simulink model "nonlinearSimulation"  (R2014a)
settings: Solver=ode4  StartTime=0.0  StopTime=50  FixedStep=.01  RelTol=1e-3
values from neighbouring files (symbols this model uses):
  C = [1 0 1 0]    [lQRdesign.m]    (also in state_space_design.m)
  g = 9.81    [energy_calc.m]    (also in lQRdesign.m; pendulum_eom.m; state_space_design.m)
  k1 = 1    [energy_calc.m]    (also in lQRdesign.m; pendulum_eom.m; state_space_design.m)
  k2 = 0.05    [energy_calc.m]    (also in lQRdesign.m; pendulum_eom.m; state_space_design.m)
  l = 1.2    [energy_calc.m]    (also in lQRdesign.m; pendulum_eom.m; state_space_design.m)
  M = 1.5    [energy_calc.m]    (also in lQRdesign.m; pendulum_eom.m; state_space_design.m)
  m = 0.5    [energy_calc.m]    (also in lQRdesign.m; pendulum_eom.m; state_space_design.m)
  sysKF = ss(A-Kf*C,[B Kf],eye(4),0*[B Kf])    [lQRdesign.m]
undefined symbols (not defined in the file or in its folder): Kr
settings Model: Creator=Mohamed Donia  LastModifiedBy=Mohamed Donia
settings DebuggingCC: AlgebraicLoopMsg=none

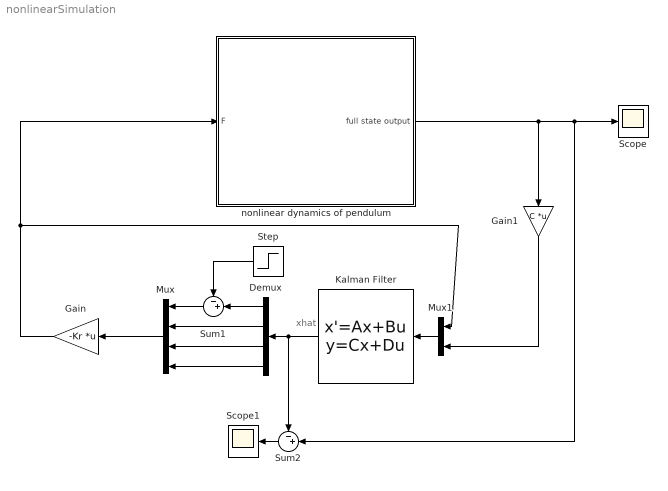
== system nonlinearSimulation ==
  note: xhat
  Demux : Demux
  Gain : Gain  Gain=-Kr  Multiplication=Matrix(K*u) (u vector)
  Gain1 : Gain  Gain=C  Multiplication=Matrix(K*u) (u vector)
  Kalman Filter : StateSpace  A=sysKF.A  B=sysKF.B  C=sysKF.C  D=sysKF.D  X0=[0 0 0 0]
  Mux : Mux
  Mux1 : Mux  Inputs=2
  Scope : Scope
  Scope1 : Scope
  Step : Step  Time=10  SampleTime=0
  Sum1 : Sum  Inputs=-+|
  Sum2 : Sum  Inputs=-+|
  nonlinear dynamics of pendulum : Subsystem
  wires:
  Kalman Filter/1 -> Sum2/1, Demux/1
  Demux/4 -> Mux/4
  Demux/3 -> Mux/3
  Demux/2 -> Mux/2
  Sum1/1 -> Mux/1
  Demux/1 -> Sum1/2
  Step/1 -> Sum1/1
  Mux/1 -> Gain/1
  Gain/1 -> nonlinear dynamics of pendulum/1(F), Mux1/1
  nonlinear dynamics of pendulum/1("full state output ") -> Sum2/2, Scope/1, Gain1/1
  Mux1/1 -> Kalman Filter/1
  Gain1/1 -> Mux1/2
  Sum2/1 -> Scope1/1

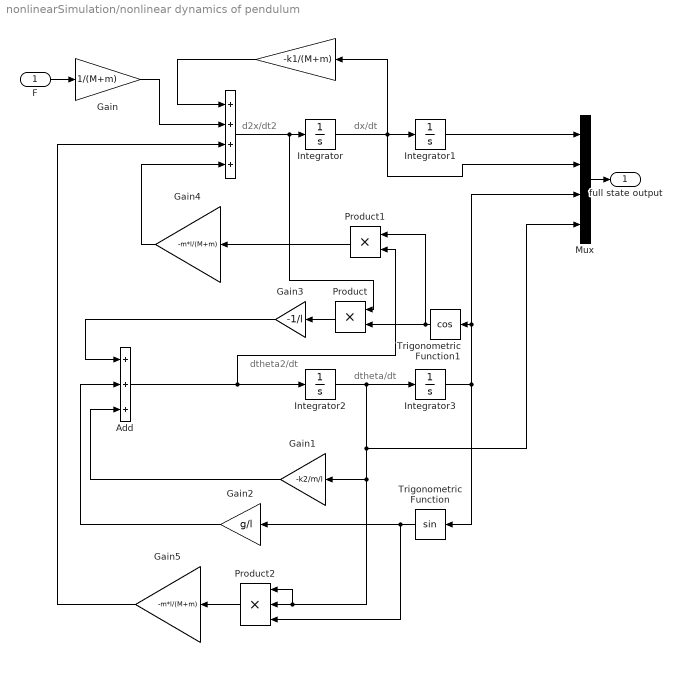
== system nonlinearSimulation/nonlinear dynamics of pendulum ==
  note: dtheta/dt
  note: dtheta2/dt
  note: dx/dt
  note: d2x/dt2
  F : Inport
  " " : Sum  Inputs=++++
  " " : Gain  Gain=-k1/(M+m)
  Add : Sum  Inputs=+++
  Gain : Gain  Gain=1/(M+m)
  Gain1 : Gain  Gain=-k2/m/l
  Gain2 : Gain  Gain=g/l
  Gain3 : Gain  Gain=-1/l
  Gain4 : Gain  Gain=-m*l/(M+m)
  Gain5 : Gain  Gain=-m*l/(M+m)
  Integrator{,1..3} (4 alike) : Integrator
  Mux : Mux
  Product : Product
  Product1 : Product
  Product2 : Product  Inputs=3
  Trigonometric Function : Trigonometry
  Trigonometric Function1 : Trigonometry  Operator=cos
  "full state output " : Outport
  wires:
  Integrator/1 -> Mux/2, " "/1, Integrator1/1
  Gain5/1 -> " "/3
  " "/1 -> Product/1, Integrator/1
  Product1/1 -> Gain4/1
  Gain3/1 -> Add/1
  Gain4/1 -> " "/4
  Product/1 -> Gain3/1
  F/1 -> Gain/1
  Gain1/1 -> Add/3
  Gain/1 -> " "/2
  Add/1 -> Product1/2, Integrator2/1
  " "/1 -> " "/1
  Integrator2/1 -> Product2/1, Product2/2, Gain1/1, Mux/4, Integrator3/1
  Product2/1 -> Gain5/1
  Trigonometric Function1/1 -> Product1/1, Product/2
  Gain2/1 -> Add/2
  Trigonometric Function/1 -> Product2/3, Gain2/1
  Integrator1/1 -> Mux/1
  Integrator3/1 -> Trigonometric Function1/1, Mux/3, Trigonometric Function/1
  Mux/1 -> "full state output "/1
